simulink model "dirdyna_walkman_robotran"  (Simulink 8.3)
settings: Solver=ode1  StartTime=0  StopTime=Tfin  FixedStep=0.0005  MaxStep=1e-2  RelTol=1e-3  AbsTol=1e-6
undefined symbols (not defined in the file or in its folder): Function_dirdynared, Modules, Robotran, S
settings Model: Creator=danilo  LastModifiedBy=danilo
settings SolverCC: InitialStep=1e-3
settings DataIOCC: SignalLoggingSaveFormat=Dataset
settings DebuggingCC: UnderspecifiedInitializationDetection=Simplified  StateNameClashWarn=none
settings GRTTargetCC: CombineOutputUpdateFcns=on  GRTInterface=off

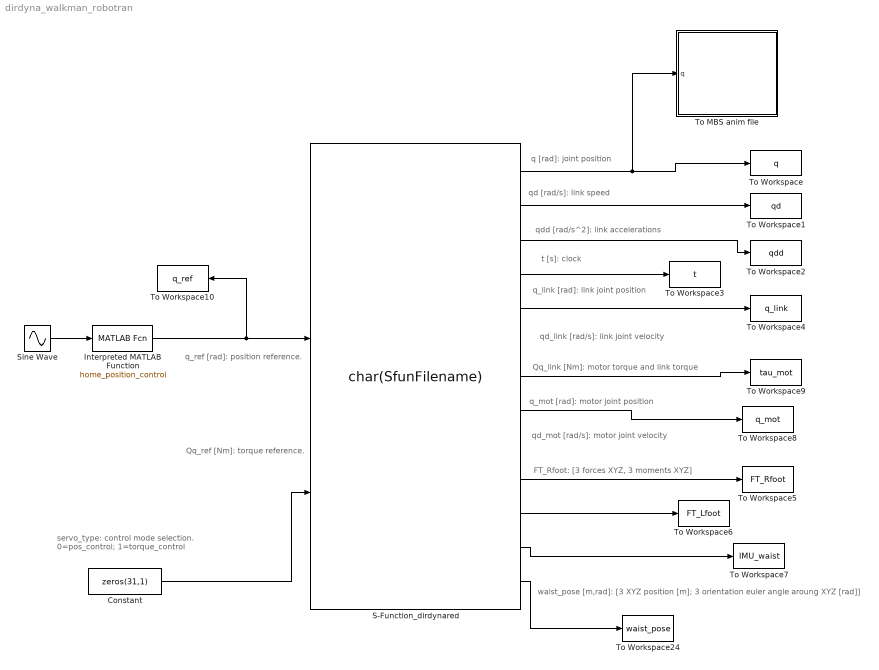
== system dirdyna_walkman_robotran ==
  note: qdd [rad/s^2]: link accelerations
  note: qd [rad/s]: link speed
  note: q [rad]: joint position
  note: t [s]: clock
  note: waist_pose [m,rad]: [3 XYZ position [m]; 3 orientation euler angle aroung XYZ [rad]]
  note: FT_Rfoot: [3 forces XYZ, 3 moments XYZ]
  note: qd_link [rad/s]: link joint velocity
  note: q_link [rad]: link joint position
  note: qd_mot [rad/s]: motor joint velocity
  note: q_mot [rad]: motor joint position
  note: Qq_link [Nm]: motor torque and link torque
  note: servo_type: control mode selection.
      | 0=pos_control; 1=torque_control
  note: q_ref [rad]: position reference.
  note: Qq_ref [Nm]: torque reference.
  Constant : Constant  Value=zeros(31,1)
  Interpreted MATLAB Function : MATLABFcn  MATLABFcn=home_position_control
  S-Function_dirdynared : S-Function  AncestorBlock=Robotran/Modules/S-Function_dirdynared  FunctionName=char(SfunFilename)  Parameters=getfield(get(gcbh,'UserData'),'mbs_data') q_ini  EnableBusSupport=off  mask(S-function: Robotran Direct Dynamics (dirdynared)){SfunFilename=mbs_sf_dirdynared_walkman_robotran, q_ini=off, creation_date=10-Mar-2016}
      mask prompts: SfunFilename "S-function filename"; q_ini "Get initial qu from block inputs"; creation_date "Enter the creation date:"
      mask help: Compute the Direct Dynamics equations using symbolic MBS formalism
      settings: OpenFcn=MBSdirdynaredSfunction
      settings: CopyFcn=|
      | MBSdirdynaredSfunction;
      | set_param(gcb,'OpenFcn','MBSdirdynaredSfunction');
      | set_param(gcb,'creation_date',date);
      | set_param(gcs,'MaxStep','1e-2');
      | set_param(gcs,'InitialStep','1e-3');
      | set_param(gcs,'RelTol','1e-3');
      | set_param(gcs,'AbsTol','1e-6');
      mask Display:
      | disp('Robotran\nDirect\nDynamics\n(dirdynared)\n-\n walkman_robotran\n-\n10-Mar-2016');
      | port_label('input',1,'Joint forces');
      | port_label('input',2,'Driven joints');
      | port_label('input',3,'q_ref');
      | port_label('input',4,'Qq_ref');
      | port_label('input',5,'servo_type');
      | port_label('input',6,'voltage');
      | port_label('output',1,'q');
      | port_label('output',2,'qd');
      | port_label('output',3,'qdd');
      | port_label('output',4,'t');
      | port_label('output',5,'q_link');
      | port_label('output',6,'qd_link');
      | port_label('output',7,'Qq_link');
      | port_label('output',8,'q_mot');
      | port_label('output',9,'qd_mot');
      | port_label('output',10,'FT_Rfoot');
      | port_label('output',11,'FT_Lfoot');
      | port_label('output',12,'IMU_waist');
      | port_label('output',13,'waist_pose');
  Sine Wave : Sin  Amplitude=0.3  Frequency=5  SampleTime=0
  To MBS anim file : Subsystem  AncestorBlock=Robotran/Utilities/To MBS anim file  StopFcn=|  mask{varname=tqres, filename=simdir.anim, overwrite=off, samplingRate=1000}
      | varname = get_param(gcb,'varname');                                     
      | filename = get_param(gcb,'filename');                                   
      | tq = evalin('base',varname);                                            
      | tt = tq.time;                                                           
      | qq = tq.signals.values;                                                 
      | % userData = get_param(gcb,'UserData');                                     
      | userData = get_param([model_name '/S-Function_dirdynared'],'UserData'); %FIX
      | mbs_data = userData.mbs_data;                                           
      | mbs_info = userData.mbs_info;                                           
      | overwrite = str2double(get_param(gcb,'overwrite'));                     
      | if isnan(overwrite)
      |     overwrite = false;
      | end
      | samplingRate = str2double(get_param(gcb,'samplingRate'));               
      | % mbs_gen_simdir(mbs_data,mbs_info,tt,qq,filename,overwrite,samplingRate);
      | mbs_gen_simdir(mbs_info.mbsname,tt,qq,filename,overwrite,samplingRate) %FIX
      mask prompts: varname "variable name"; filename "anim file name"; overwrite "overwrite flag"; samplingRate "sampling rate"
      settings: CopyFcn=MBStoAnimFile_v2;  OpenFcn=MBStoAnimFile_v2;
      mask Display: image(imread('Logo_anim.jpg'))
  To Workspace : ToWorkspace  VariableName=q  SampleTime=-1
  To Workspace1 : ToWorkspace  VariableName=qd  SampleTime=-1
  To Workspace10 : ToWorkspace  VariableName=q_ref  SampleTime=-1
  To Workspace2 : ToWorkspace  VariableName=qdd  SampleTime=-1
  To Workspace24 : ToWorkspace  VariableName=waist_pose  SampleTime=-1
  To Workspace3 : ToWorkspace  VariableName=t  SampleTime=-1
  To Workspace4 : ToWorkspace  VariableName=q_link  SampleTime=-1
  To Workspace5 : ToWorkspace  VariableName=FT_Rfoot  SampleTime=-1
  To Workspace6 : ToWorkspace  VariableName=FT_Lfoot  SampleTime=-1
  To Workspace7 : ToWorkspace  VariableName=IMU_waist  SampleTime=-1
  To Workspace8 : ToWorkspace  VariableName=q_mot  SampleTime=-1
  To Workspace9 : ToWorkspace  VariableName=tau_mot  SampleTime=-1
  wires:
  Constant/1 -> S-Function_dirdynared/5
  S-Function_dirdynared/1 -> To MBS anim file/1(q), To Workspace/1
  S-Function_dirdynared/2 -> To Workspace1/1
  S-Function_dirdynared/3 -> To Workspace2/1
  S-Function_dirdynared/4 -> To Workspace3/1
  S-Function_dirdynared/11 -> To Workspace6/1
  S-Function_dirdynared/12 -> To Workspace7/1
  S-Function_dirdynared/8 -> To Workspace8/1
  S-Function_dirdynared/7 -> To Workspace9/1
  Sine Wave/1 -> Interpreted MATLAB Function/1
  S-Function_dirdynared/10 -> To Workspace5/1
  S-Function_dirdynared/13 -> To Workspace24/1
  Interpreted MATLAB Function/1 -> S-Function_dirdynared/3, To Workspace10/1
  S-Function_dirdynared/5 -> To Workspace4/1

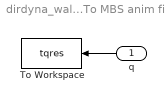
== system dirdyna_walkman_robotran/To MBS anim file ==
  q : Inport
  To Workspace : ToWorkspace  VariableName=tqres  SaveFormat=Structure With Time  SampleTime=-1
  wires:
  q/1 -> To Workspace/1
